simulink model "trajectory_planner"  (R2015b)
settings: Solver=ode45  SolverMode=SingleTasking  StartTime=0.0  StopTime=10  RelTol=1e-3
values from neighbouring files (symbols this model uses):
  a_max = 543    [workshopB.m]
  F_c = 1.5e-3    (= 0.0015)    [t3s.m]    (also in workshopB.m)
  J1 = 6e-4    (= 0.0006)    [ControllerC.m]    (also in t3s.m; workshopB.m)
  motor = motor_pars    [t3s.m]    (also in workshopB.m)
  n = 5    [ControllerC.m]    (also in t3s.m; workshopB.m)
  R_vector_p = [1 r0 0]    [workshopB.m]
  S_vector_p = [s2 s1 s0]    [workshopB.m]
  v_max = 230    [workshopB.m]
libraries: simulink x1
settings Model: Creator=Gabriel  LastModifiedBy=gabri
settings SolverCC: ZeroCrossAlgorithm=Adaptive
settings DataIOCC: SaveFormat=Array
settings OptimizationCC: BlockReduction=off  BooleanDataType=off
settings DebuggingCC: SaveWithParameterizedLinksMsg=none  UnderspecifiedInitializationDetection=Classic  MergeDetectMultiDrivingBlocksExec=none  SignalResolutionControl=TryResolveAllWithWarning
settings HardwareCC: ProdBitPerPointer=32  ProdLargestAtomicFloat=None  ProdIntDivRoundTo=Undefined  ProdEndianess=Unspecified  ProdWordSize=32  ProdHWDeviceType=32-bit Generic  TargetBitPerPointer=64  TargetLongLongMode=on  TargetIntDivRoundTo=Zero  TargetEndianess=LittleEndian  TargetWordSize=64  TargetHWDeviceType=MATLAB Host  ProdEqTarget=off
settings GRTTargetCC: GeneratePreprocessorConditionals=Disable all
settings ConfigComp: CovModelRefEnable=Off  CovSFcnEnable=off

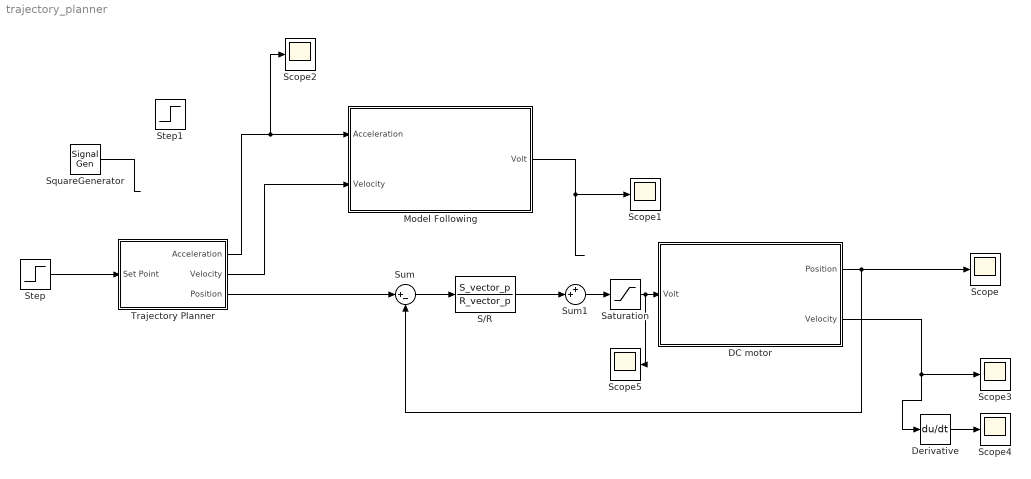
== system trajectory_planner ==
  DC motor : Subsystem
  Derivative : Derivative
  Model Following : Subsystem
  S/R : TransferFcn  Numerator=S_vector_p  Denominator=R_vector_p
  Saturation : Saturate  UpperLimit=24  LowerLimit=-24
  Scope{,1..5} (6 alike) : Scope
  SquareGenerator : SignalGenerator  WaveForm=square  Amplitude=10  Units=rad/sec
  Step : Step  Time=0  After=10  SampleTime=0
  Step1 : Step  Time=0  After=50  SampleTime=0
  Sum : Sum  Inputs=|+-
  Sum1 : Sum  Inputs=++|
  Trajectory Planner : Subsystem
  wires:
  Step/1 -> Trajectory Planner/1(Set Point)
  Sum/1 -> S/R/1
  DC motor/1(Position) -> Scope/1, Sum/2
  S/R/1 -> Sum1/2
  Model Following/1(Volt) -> Scope1/1
  SquareGenerator/1 -> ?
  Trajectory Planner/3(Position) -> Sum/1
  Trajectory Planner/1(Acceleration) -> Scope2/1, Model Following/1("Acceleration ")
  Trajectory Planner/2(Velocity) -> Model Following/2(Velocity)
  DC motor/2(Velocity) -> Derivative/1, Scope3/1
  Derivative/1 -> Scope4/1
  Sum1/1 -> Saturation/1
  Saturation/1 -> Scope5/1, DC motor/1(Volt)

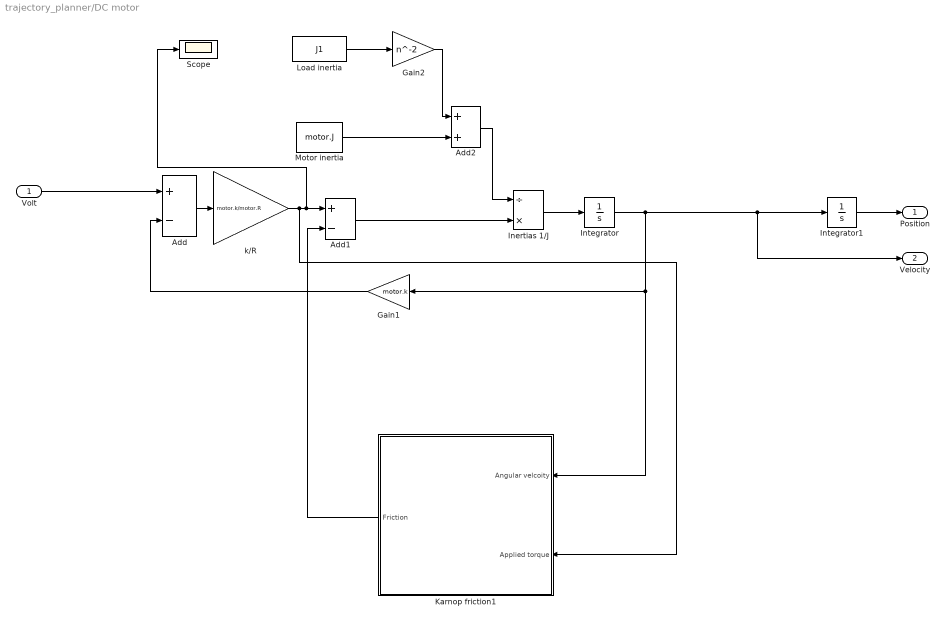
== system trajectory_planner/DC motor ==
  Volt : Inport
  Add : Sum  Inputs=+-
  Add1 : Sum  Inputs=+-
  Add2 : Sum
  Gain1 : Gain  Gain=motor.k
  Gain2 : Gain  Gain=n^-2
  Inertias 1/J : Product  Inputs=/*
  Integrator : Integrator
  Integrator1 : Integrator
  Karnop friction1 : Subsystem
  Load inertia : Constant  Value=J1
  Motor inertia : Constant  Value=motor.J
  Scope : Scope
  "k/R " : Gain  Gain=motor.k/motor.R
  Position : Outport
  Velocity : Outport  Port=2
  wires:
  Karnop friction1/1(Friction) -> Add1/2
  Add2/1 -> Inertias 1/J/1
  Gain2/1 -> Add2/1
  Load inertia/1 -> Gain2/1
  Motor inertia/1 -> Add2/2
  Integrator/1 -> Integrator1/1, Velocity/1, Karnop friction1/1(Angular velcoity), Gain1/1
  Volt/1 -> Add/1
  Add1/1 -> Inertias 1/J/2
  Integrator1/1 -> Position/1
  Inertias 1/J/1 -> Integrator/1
  "k/R "/1 -> Scope/1, Add1/1, Karnop friction1/2(Applied torque)
  Add/1 -> "k/R "/1
  Gain1/1 -> Add/2

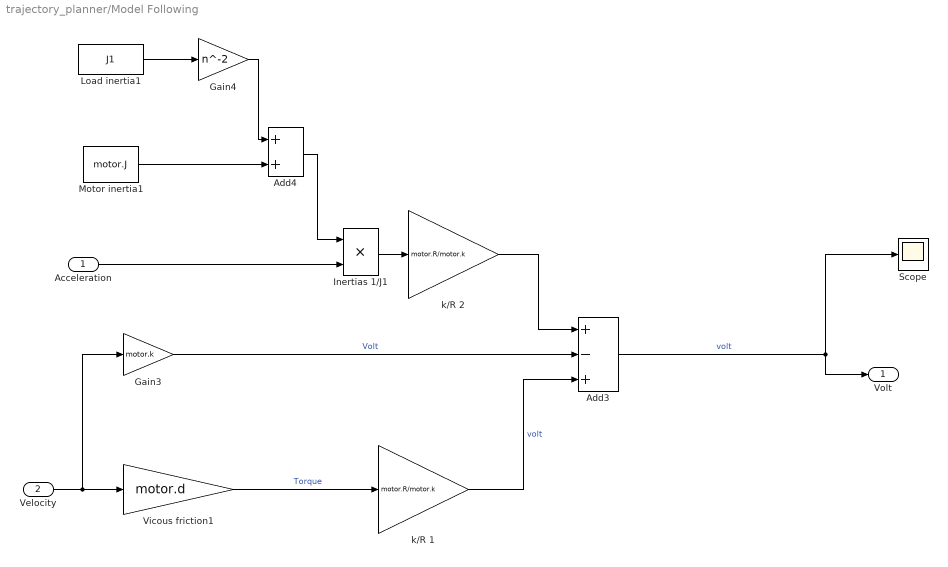
== system trajectory_planner/Model Following ==
  "Acceleration " : Inport
  Velocity : Inport  Port=2
  Add3 : Sum  Inputs=+-+
  Add4 : Sum
  Gain3 : Gain  Gain=motor.k
  Gain4 : Gain  Gain=n^-2
  Inertias 1/J1 : Product  Inputs=**
  Load inertia1 : Constant  Value=J1
  Motor inertia1 : Constant  Value=motor.J
  Scope : Scope
  Vicous friction1 : Gain  Gain=motor.d
  k/R 1 : Gain  Gain=motor.R/motor.k
  k/R 2 : Gain  Gain=motor.R/motor.k
  Volt : Outport
  wires:
  Velocity/1 -> Gain3/1, Vicous friction1/1
  Vicous friction1/1 -> k/R 1/1  "Torque"
  Gain3/1 -> Add3/2  "Volt"
  k/R 1/1 -> Add3/3  "volt"
  Add3/1 -> Volt/1, Scope/1  "volt"
  Motor inertia1/1 -> Add4/2
  Load inertia1/1 -> Gain4/1
  Gain4/1 -> Add4/1
  Add4/1 -> Inertias 1/J1/1
  "Acceleration "/1 -> Inertias 1/J1/2
  Inertias 1/J1/1 -> k/R 2/1
  k/R 2/1 -> Add3/1

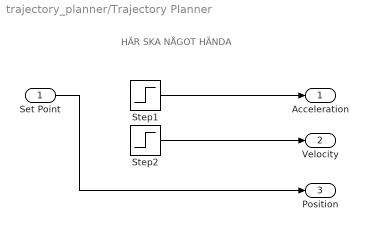
== system trajectory_planner/Trajectory Planner ==
  note: HÄR SKA NÅGOT HÄNDA
  Set Point : Inport
  Step1 : Step  Time=0  After=a_max  SampleTime=0
  Step2 : Step  Time=0  After=v_max  SampleTime=0
  Acceleration : Outport
  Velocity : Outport  Port=2
  Position : Outport  Port=3
  wires:
  Set Point/1 -> Position/1
  Step2/1 -> Velocity/1
  Step1/1 -> Acceleration/1

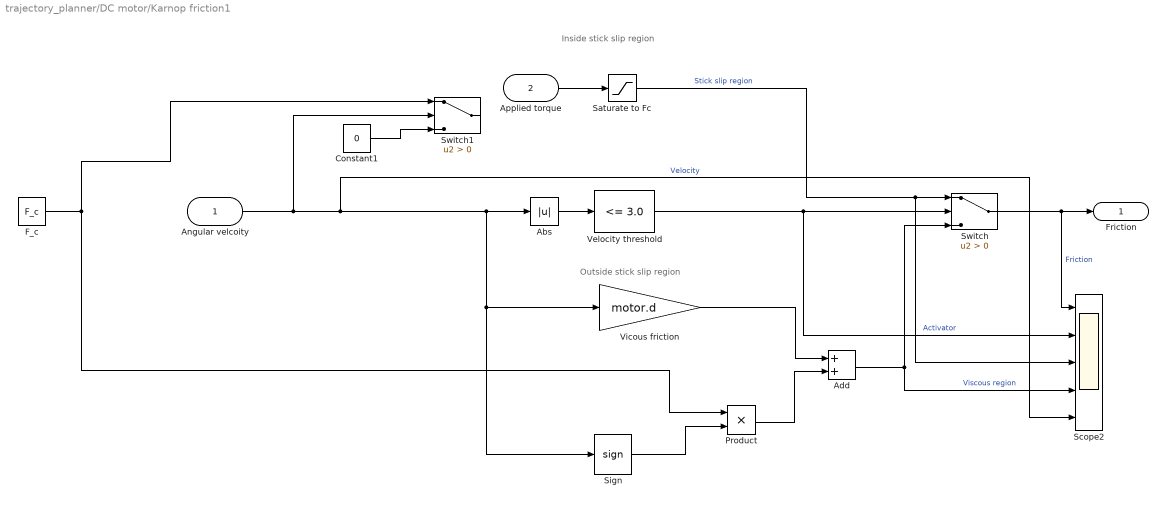
== system trajectory_planner/DC motor/Karnop friction1 ==
  note: Outside stick slip region
  note: Inside stick slip region
  Angular velcoity : Inport
  Applied torque : Inport  Port=2
  Abs : Abs  ZeroCross=off
  Add : Sum
  Constant1 : Constant  Value=0
  F_c : Constant  Value=F_c
  Product : Product
  Saturate to Fc : Saturate  UpperLimit=F_c  LowerLimit=-F_c  ZeroCross=off
  Scope2 : Scope  NumInputPorts=5
  Sign : Signum  ZeroCross=off
  Switch : Switch  Criteria=u2 > Threshold  ZeroCross=off
  Switch1 : Switch  Criteria=u2 > Threshold  ZeroCross=off
  "Velocity threshold " : simulink/Logic and Bit Operations/Compare To Constant  relop=<=  const=3.0  OutDataTypeStr=boolean
  Vicous friction : Gain  Gain=motor.d
  Friction : Outport
  wires:
  Applied torque/1 -> Saturate to Fc/1
  Add/1 -> Scope2/4, Switch/3  "Viscous region"
  Sign/1 -> Product/2
  F_c/1 -> Product/1, Switch1/1
  Vicous friction/1 -> Add/1
  Product/1 -> Add/2
  Abs/1 -> "Velocity threshold "/1
  "Velocity threshold "/1 -> Switch/2, Scope2/2  "Activator"
  Angular velcoity/1 -> Switch1/2, Sign/1, Vicous friction/1, Abs/1, Scope2/5  "Velocity"
  Switch/1 -> Friction/1, Scope2/1  "Friction"
  Saturate to Fc/1 -> Switch/1, Scope2/3  "Stick slip region"
  Constant1/1 -> Switch1/3
